simulink model "Rishi_Rajasekhar_Industrial_Temperature_Control_Simulation"  (R2024b)
settings: Solver=ode45  StartTime=0.0  StopTime=50  MaxStep=0.01  RelTol=1e-6  AbsTol=1e-8
libraries: slpidlib x1
settings Model: Creator=Rishi  LastModifiedBy=Rishi

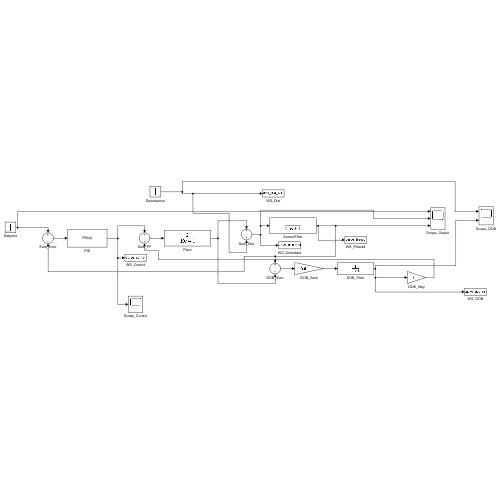
[thumbnail: Simulink's stored preview of the top-level diagram]
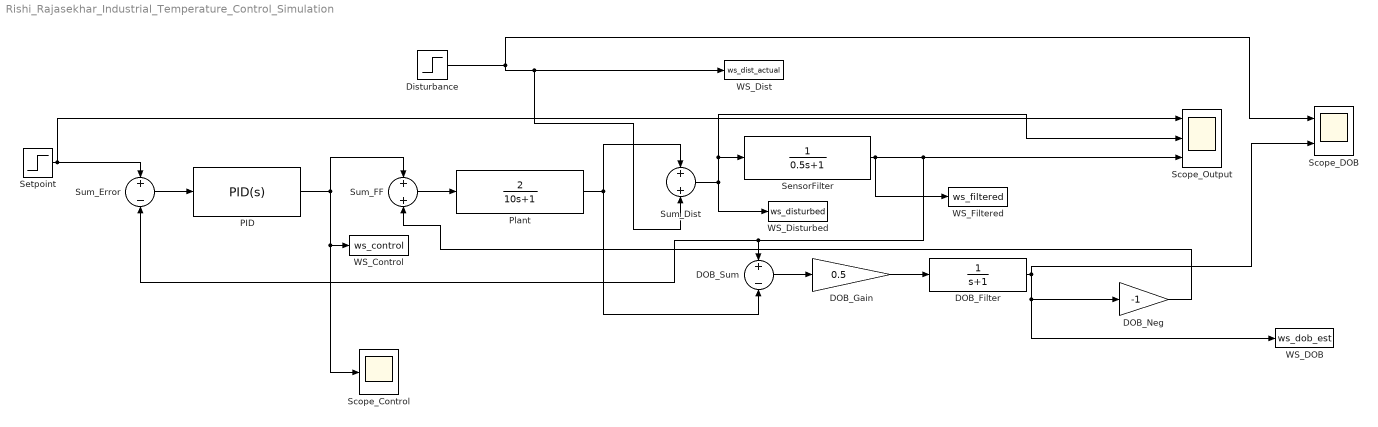
== system Rishi_Rajasekhar_Industrial_Temperature_Control_Simulation ==
  DOB_Filter : TransferFcn  Numerator=1  Denominator=[1 1]
  DOB_Gain : Gain  Gain=0.5
  DOB_Neg : Gain  Gain=-1
  DOB_Sum : Sum  Inputs=+-
  Disturbance : Step  Time=15  After=-0.25  SampleTime=0
  PID : slpidlib/PID Controller  Controller=PID  Form=Parallel  TimeDomain=Continuous-time  UseExternalTs=off  SampleTime=-1  IntegratorMethod=Forward Euler  FilterMethod=Forward Euler  ControllerParametersSource=internal  P=2.5  I=0.35  UseKiTs=off  D=0.8  UseExternalDerivativeSource=off  N=10  UseFilter=on  TunerSelectOption=Transfer Function Based (PID Tuner App)  InitialConditionSource=internal  InitialConditionForIntegrator=0  InitialConditionForFilter=0  DifferentiatorICPrevScaledInput=0  ExternalReset=none  TrackingMode=off  Kt=1  LimitOutput=off  SatLimitsSource=internal  UpperSaturationLimit=inf  LowerSaturationLimit=-inf  LinearizeAsGain=on  AntiWindupMode=none  Kb=1  LimitIntegrator=off  UpperIntegratorSaturationLimit=inf  LowerIntegratorSaturationLimit=-inf  POutMin=[]  POutMax=[]  IOutMin=[]  IOutMax=[]  DOutMin=[]  DOutMax=[]  NOutMin=[]  NOutMax=[]  SumOutMin=[]  SumOutMax=[]  SaturationOutMin=[]  SaturationOutMax=[]  PParamMin=[]  PParamMax=[]  IParamMin=[]  IParamMax=[]  DParamMin=[]  DParamMax=[]  NParamMin=[]  NParamMax=[]  KbParamMin=[]  KbParamMax=[]  KtParamMin=[]  KtParamMax=[]  KbOutMin=[]  KbOutMax=[]  KtOutMin=[]  KtOutMax=[]  IntegratorOutMin=[]  IntegratorOutMax=[]  FilterOutMin=[]  FilterOutMax=[]  SumI1OutMin=[]  SumI1OutMax=[]  SumI2OutMin=[]  SumI2OutMax=[]  SumI3OutMin=[]  SumI3OutMax=[]  SumI4OutMin=[]  SumI4OutMax=[]  SumDOutMin=[]  SumDOutMax=[]  DifferentiatorOutMin=[]  DifferentiatorOutMax=[]  FilterDiffOutCoefMin=[]  FilterDiffOutCoefMax=[]  ReciprocalOutMin=[]  ReciprocalOutMax=[]  SumDenOutMin=[]  SumDenOutMax=[]  SumNumOutMin=[]  SumNumOutMax=[]  DivideOutMin=[]  DivideOutMax=[]  UdiffTsProdOutMin=[]  UdiffTsProdOutMax=[]  NTsProdOutMin=[]  NTsProdOutMax=[]  UintegralTsProdOutMin=[]  UintegralTsProdOutMax=[]  UngainTsProdOutMin=[]  UngainTsProdOutMax=[]  ClampingZeroOutDataTypeStr=Inherit: Inherit via back propagation  ClampingZeroOutMin=[]  ClampingZeroOutMax=[]  FilterDenConstantOutDataTypeStr=Inherit: Inherit via back propagation  FilterDenConstantOutMin=[]  FilterDenConstantOutMax=[]  PCopyOutDataTypeStr=Inherit: Inherit via back propagation  PCopyOutMin=[]  PCopyOutMax=[]  NCopyOutDataTypeStr=Inherit: Inherit via back propagation  NCopyOutMin=[]  NCopyOutMax=[]  IntegratorContinuousStateAttributes=''  IntegratorStateMustResolveToSignalObject=off  IntegratorRTWStateStorageClass=Auto  FilterContinuousStateAttributes=''  FilterStateMustResolveToSignalObject=off  FilterRTWStateStorageClass=Auto  ParallelPVariant=InternalParameters  IdealPVariant=Disabled  IVariant=InternalParameters  DVariant=InternalParameters  IntegratorVariant=Continuous  SatVariant=Disabled  AWVariant=Passthrough  PCopyVariant=Disabled  TRVariant=Disabled  FdbkBlocksVariant=Forward  IdealPFdbkVariant=Disabled  SatFdbkVariant=Disabled  DerivativeFilterVariant=ContFilter  NVariant=InternalParameters  NCopyVariant=Disabled  FilterICVariant=InternalICsFilter  IntegratorICVariant=InternalICs  ExternalResetVariant=Disabled  TRSumVariant=Passthrough  SumFdbkVariant=Disabled  SumVariant=Sum_PID  TsampFilterVariant=InternalTs  TsampNgainVariant=Passthrough  TsampIntegralVariant=Disabled_SignalSpec  ExternalSaturationOutDataTypeStr=Inherit: Same as second input  DerivativeSourceVariant=ErrorSignal  PreIntVariant=InternalPreInt
  Plant : TransferFcn  Numerator=2  Denominator=[10 1]
  Scope_Control : Scope
  Scope_DOB : Scope  NumInputPorts=2
  Scope_Output : Scope  NumInputPorts=3
  SensorFilter : TransferFcn  Numerator=1  Denominator=[0.5 1]
  Setpoint : Step  Time=0  SampleTime=0
  Sum_Dist : Sum
  Sum_Error : Sum  Inputs=+-
  Sum_FF : Sum
  WS_Control : ToWorkspace  VariableName=ws_control  SaveFormat=Timeseries  SampleTime=-1
  WS_DOB : ToWorkspace  VariableName=ws_dob_est  SaveFormat=Timeseries  SampleTime=-1
  WS_Dist : ToWorkspace  VariableName=ws_dist_actual  SaveFormat=Timeseries  SampleTime=-1
  WS_Disturbed : ToWorkspace  VariableName=ws_disturbed  SaveFormat=Timeseries  SampleTime=-1
  WS_Filtered : ToWorkspace  VariableName=ws_filtered  SaveFormat=Timeseries  SampleTime=-1
  wires:
  Setpoint/1 -> Sum_Error/1, Scope_Output/1
  Sum_Error/1 -> PID/1
  PID/1 -> Sum_FF/1, Scope_Control/1, WS_Control/1
  Sum_FF/1 -> Plant/1
  Plant/1 -> Sum_Dist/1, DOB_Sum/2
  Disturbance/1 -> Scope_DOB/1, Sum_Dist/2, WS_Dist/1
  Sum_Dist/1 -> Scope_Output/2, SensorFilter/1, WS_Disturbed/1
  SensorFilter/1 -> Scope_Output/3, Sum_Error/2, DOB_Sum/1, WS_Filtered/1
  DOB_Sum/1 -> DOB_Gain/1
  DOB_Gain/1 -> DOB_Filter/1
  DOB_Filter/1 -> WS_DOB/1, DOB_Neg/1, Scope_DOB/2
  DOB_Neg/1 -> Sum_FF/2
